simulink library "rwa_rpm_to_body_momentum"  (R2018b)
settings: Solver=VariableStepAuto  StartTime=0.0  StopTime=10.0  RelTol=1e-3
undefined symbols (not defined in the file or in its folder): fswParams
settings Model: Creator=aact_  LastModifiedBy=aact_

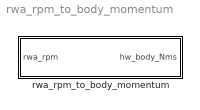
== system rwa_rpm_to_body_momentum ==
  rwa_rpm_to_body_momentum : Subsystem  TreatAsAtomicUnit=on
      settings: RTWFcnNameOpts=Use subsystem name  RTWFileNameOpts=Use subsystem name

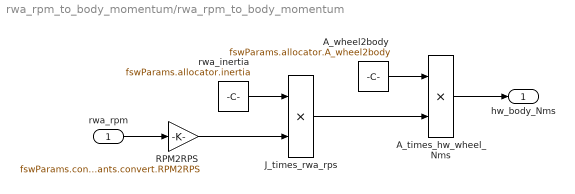
== system rwa_rpm_to_body_momentum/rwa_rpm_to_body_momentum ==
  rwa_rpm : Inport
  A_times_hw_wheel_Nms : Product
  A_wheel2body : Constant  Value=fswParams.allocator.A_wheel2body
  J_times_rwa_rps : Product
  RPM2RPS : Gain  Gain=fswParams.constants.convert.RPM2RPS
  rwa_inertia : Constant  Value=fswParams.allocator.inertia
  hw_body_Nms : Outport
  wires:
  rwa_rpm/1 -> RPM2RPS/1
  RPM2RPS/1 -> J_times_rwa_rps/2
  rwa_inertia/1 -> J_times_rwa_rps/1
  J_times_rwa_rps/1 -> A_times_hw_wheel_Nms/2
  A_times_hw_wheel_Nms/1 -> hw_body_Nms/1
  A_wheel2body/1 -> A_times_hw_wheel_Nms/1
